simulink model "Problema_2_incremental"  (R2014a)
settings: Solver=ode45  StartTime=0.0  StopTime=10.0  RelTol=1e-3
values from neighbouring files (symbols this model uses):
  b = 0.5    [Problema_2_tp2_variables.m]
  ki = (2 * ieq * k)/yeq    (= 7.8400627205)    [Problema_2_tp2_variables.m]
  ky = -(k * ieq^2)/yeq^2    (= -7.68332293268)    [Problema_2_tp2_variables.m]
  L = 0.01    [Problema_2_tp2_variables.m]
  M = 0.2    [Problema_2_tp2_variables.m]
  R = 20    [Problema_2_tp2_variables.m]
settings Model: Creator=lraff  LastModifiedBy=lraff

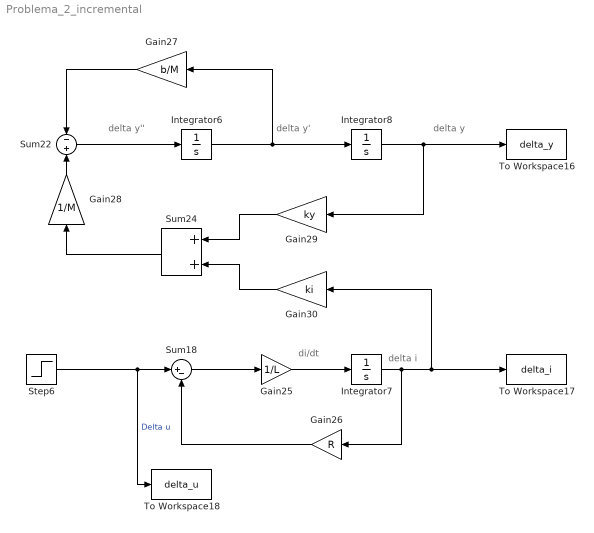
== system Problema_2_incremental ==
  note: di/dt
  note: delta i
  note: delta y''
  note: delta y'
  note: delta y
  Gain25 : Gain  Gain=1/L
  Gain26 : Gain  Gain=R
  Gain27 : Gain  Gain=b/M
  Gain28 : Gain  Gain=1/M
  Gain29 : Gain  Gain=ky
  Gain30 : Gain  Gain=ki
  Integrator6 : Integrator
  Integrator7 : Integrator
  Integrator8 : Integrator
  Step6 : Step  After=0.2  SampleTime=0
  Sum18 : Sum  Inputs=|+-
  Sum22 : Sum  Inputs=-|+
  Sum24 : Sum
  To Workspace16 : ToWorkspace  VariableName=delta_y  SaveFormat=Timeseries  SampleTime=-1
  To Workspace17 : ToWorkspace  VariableName=delta_i  SaveFormat=Timeseries  SampleTime=-1
  To Workspace18 : ToWorkspace  VariableName=delta_u  SaveFormat=Timeseries  SampleTime=-1
  wires:
  Sum18/1 -> Gain25/1
  Gain25/1 -> Integrator7/1
  Gain26/1 -> Sum18/2
  Sum22/1 -> Integrator6/1
  Integrator6/1 -> Gain27/1, Integrator8/1
  Gain27/1 -> Sum22/1
  Step6/1 -> To Workspace18/1, Sum18/1  "Delta u"
  Integrator8/1 -> Gain29/1, To Workspace16/1
  Gain29/1 -> Sum24/1
  Integrator7/1 -> Gain30/1, To Workspace17/1, Gain26/1
  Gain30/1 -> Sum24/2
  Sum24/1 -> Gain28/1
  Gain28/1 -> Sum22/2
